simulink model "mrefrobotarm_modified_previous_y_error_previous_u"  (R2018b)
settings: Solver=FixedStepAuto  StartTime=0.0  StopTime=60  RelTol=1e-3  AbsTol=1e-6
undefined symbols (not defined in the file or in its folder): now, sfunxy2, simin
libraries: neural x368, simulink x1
(part 3 of 10)

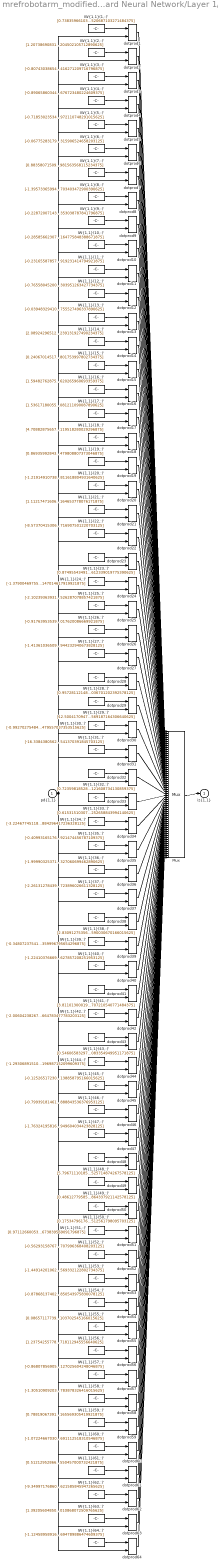
== system mrefrobotarm_modified_previous_y_error_previous_u/Feed-Forward Neural Network/Layer 1/IW{1,1} ==
  "pd{1,1}" : Inport  PortDimensions=7
      mask Display: e = 0.06;c1 = [120 230 180]/255;c2 = ([120 230 180]+0)/(256+128);c3 = ([120 230 180]+128)/(256+128);patch([0 1 1 0],[0 0 1 1],c1);patch([0 1 1 1-e 1-e 0+e],[0 0 1 1-e 0+e 0+e],c2);patch([0 0 1 1-e 0+e 0+e],[0 1 1 1-e 1-e 0+e],c3);plot([0 1 1 0 0],[0 0 1 1 0]);
  "IW{1,1}(1,:)'" : Constant  Value=[0.73835966103695149787000673313741572201251983642578125;-0.94961190463521660820589431750704534351825714111328125;1.6035911924959707075544201870798133313655853271484375;1.2440476828636082284873509706812910735607147216796875;-1.3632517507492050157225094153545796871185302734375;-0.5284581869871158854579107355675660073757171630859375;0.17161240081002249180386343141435645520687103271484375]
      mask Display: e = 0.06;c1 = [120 150 230]/255;c2 = ([120 150 230]+0)/383;c3 = ([120 150 230]+128)/383;patch([0 1 1 0],[0 0 1 1],c1);patch([0 1 1 1-e 1-e 0+e],[0 0 1 1-e 0+e 0+e],c2);patch([0 0 1 1-e 0+e 0+e],[0 1 1 1-e 1-e 0+e],c3);plot([0 1 1 0 0],[0 0 1 1 0]);disp('Weights');
  "IW{1,1}(10,:)'" : Constant  Value=[-0.285856623070984305901021116369520314037799835205078125;0.2344776406677883950901986054304870776832103729248046875;-1.315520776721690321409141688491217792034149169921875;1.074880530465292860498038862715475261211395263671875;-2.319666095832283669864182229503057897090911865234375;0.6986740963338966547979680399294011294841766357421875;-0.300490225799896648606335247677634470164775848388671875]
      mask Display: e = 0.06;c1 = [120 150 230]/255;c2 = ([120 150 230]+0)/383;c3 = ([120 150 230]+128)/383;patch([0 1 1 0],[0 0 1 1],c1);patch([0 1 1 1-e 1-e 0+e],[0 0 1 1-e 0+e 0+e],c2);patch([0 0 1 1-e 0+e 0+e],[0 1 1 1-e 1-e 0+e],c3);plot([0 1 1 0 0],[0 0 1 1 0]);disp('Weights');
  "IW{1,1}(11,:)'" : Constant  Value=[-0.2316558785704640743841054018048453144729137420654296875;0.69436199539330900609712671212037093937397003173828125;0.0092057493650668266449432763920412980951368808746337890625;1.1913003539647768480591594197903759777545928955078125;0.329665431400123776217725435344618745148181915283203125;-0.03705915414620364334297164532472379505634307861328125;-2.367396266890927858383975035394541919231414794921875]
      mask Display: e = 0.06;c1 = [120 150 230]/255;c2 = ([120 150 230]+0)/383;c3 = ([120 150 230]+128)/383;patch([0 1 1 0],[0 0 1 1],c1);patch([0 1 1 1-e 1-e 0+e],[0 0 1 1-e 0+e 0+e],c2);patch([0 0 1 1-e 0+e 0+e],[0 1 1 1-e 1-e 0+e],c3);plot([0 1 1 0 0],[0 0 1 1 0]);disp('Weights');
  "IW{1,1}(12,:)'" : Constant  Value=[-0.76558045200224367210495302060735411942005157470703125;-1.3880666042352911571100548826507292687892913818359375;1.240281466247820763015852207900024950504302978515625;-0.0943438152588715051027890012846910394728183746337890625;-1.1016339629113909293067763428553007543087005615234375;0.77645097802456730651243788088322617113590240478515625;1.0157545017459932434888969510211609303951263427734375]
      mask Display: e = 0.06;c1 = [120 150 230]/255;c2 = ([120 150 230]+0)/383;c3 = ([120 150 230]+128)/383;patch([0 1 1 0],[0 0 1 1],c1);patch([0 1 1 1-e 1-e 0+e],[0 0 1 1-e 0+e 0+e],c2);patch([0 0 1 1-e 0+e 0+e],[0 1 1 1-e 1-e 0+e],c3);plot([0 1 1 0 0],[0 0 1 1 0]);disp('Weights');
  "IW{1,1}(13,:)'" : Constant  Value=[-0.0394832941047644492282842065833392553031444549560546875;0.2683433283804415037110402408870868384838104248046875;-1.9772412570219646266167501380550675094127655029296875;-1.3369533766644858818750662976526655256748199462890625;0.383848968826891734362760644216905348002910614013671875;-0.82866232479277546207896421037730760872364044189453125;-0.71448374375757206511394770132028497755527496337890625]
      mask Display: e = 0.06;c1 = [120 150 230]/255;c2 = ([120 150 230]+0)/383;c3 = ([120 150 230]+128)/383;patch([0 1 1 0],[0 0 1 1],c1);patch([0 1 1 1-e 1-e 0+e],[0 0 1 1-e 0+e 0+e],c2);patch([0 0 1 1-e 0+e 0+e],[0 1 1 1-e 1-e 0+e],c3);plot([0 1 1 0 0],[0 0 1 1 0]);disp('Weights');
  "IW{1,1}(14,:)'" : Constant  Value=[2.089242965128133899810336515656672418117523193359375;1.0583956137306387290664133615791797637939453125;1.2221961841086137479095441449317149817943572998046875;-0.9640381765065815233839430220541544258594512939453125;2.007169466431919513382808872847817838191986083984375;-0.005116273422281165071667796695464858203195035457611083984375;0.5419457531010729578468954059644602239131927490234375]
      mask Display: e = 0.06;c1 = [120 150 230]/255;c2 = ([120 150 230]+0)/383;c3 = ([120 150 230]+128)/383;patch([0 1 1 0],[0 0 1 1],c1);patch([0 1 1 1-e 1-e 0+e],[0 0 1 1-e 0+e 0+e],c2);patch([0 0 1 1-e 0+e 0+e],[0 1 1 1-e 1-e 0+e],c3);plot([0 1 1 0 0],[0 0 1 1 0]);disp('Weights');
  "IW{1,1}(15,:)'" : Constant  Value=[0.240670145172809435418770362957729957997798919677734375;-0.37262437066721532108459769006003625690937042236328125;0.7519452971248181682994982111267745494842529296875;-0.43618047326959208387364697045995853841304779052734375;-2.164127657796442338877795918961055576801300048828125;-1.4690578945890966355847240265575237572193145751953125;1.03041595327624602163041345193050801753997802734375]
      mask Display: e = 0.06;c1 = [120 150 230]/255;c2 = ([120 150 230]+0)/383;c3 = ([120 150 230]+128)/383;patch([0 1 1 0],[0 0 1 1],c1);patch([0 1 1 1-e 1-e 0+e],[0 0 1 1-e 0+e 0+e],c2);patch([0 0 1 1-e 0+e 0+e],[0 1 1 1-e 1-e 0+e],c3);plot([0 1 1 0 0],[0 0 1 1 0]);disp('Weights');
  "IW{1,1}(16,:)'" : Constant  Value=[1.594827628756812831767319948994554579257965087890625;-0.409790418491936481171222794728237204253673553466796875;0.5354336553033169909809885211871005594730377197265625;0.293245297642927560399783715183730237185955047607421875;-1.1159358132358245807580487962695769965648651123046875;0.6919927373218188737524769749143160879611968994140625;-1.12512451883200181868005529395304620265960693359375]
      mask Display: e = 0.06;c1 = [120 150 230]/255;c2 = ([120 150 230]+0)/383;c3 = ([120 150 230]+128)/383;patch([0 1 1 0],[0 0 1 1],c1);patch([0 1 1 1-e 1-e 0+e],[0 0 1 1-e 0+e 0+e],c2);patch([0 0 1 1-e 0+e 0+e],[0 1 1 1-e 1-e 0+e],c3);plot([0 1 1 0 0],[0 0 1 1 0]);disp('Weights');
  "IW{1,1}(17,:)'" : Constant  Value=[1.536171800559593680901571133290417492389678955078125;0.044760026132134471399393049750869977287948131561279296875;0.6869129687880015655565557608497329056262969970703125;0.475311403464723836176375471040955744683742523193359375;0.429599864159958599874045148681034334003925323486328125;2.369256087953004907831200398504734039306640625;0.80062373149870647015546865077340044081211090087890625]
      mask Display: e = 0.06;c1 = [120 150 230]/255;c2 = ([120 150 230]+0)/383;c3 = ([120 150 230]+128)/383;patch([0 1 1 0],[0 0 1 1],c1);patch([0 1 1 1-e 1-e 0+e],[0 0 1 1-e 0+e 0+e],c2);patch([0 0 1 1-e 0+e 0+e],[0 1 1 1-e 1-e 0+e],c3);plot([0 1 1 0 0],[0 0 1 1 0]);disp('Weights');
  "IW{1,1}(18,:)'" : Constant  Value=[4.70882875657937471913783156196586787700653076171875;1.0182941971839178929570834952755831182003021240234375;-0.29646960125124144358466082849190570414066314697265625;-2.63562093522858020833155023865401744842529296875;1.25983914696097176744160606176592409610748291015625;0.8392764608202714082807460727053694427013397216796875;0.38937859950317121882079618444549851119518280029296875]
      mask Display: e = 0.06;c1 = [120 150 230]/255;c2 = ([120 150 230]+0)/383;c3 = ([120 150 230]+128)/383;patch([0 1 1 0],[0 0 1 1],c1);patch([0 1 1 1-e 1-e 0+e],[0 0 1 1-e 0+e 0+e],c2);patch([0 0 1 1-e 0+e 0+e],[0 1 1 1-e 1-e 0+e],c3);plot([0 1 1 0 0],[0 0 1 1 0]);disp('Weights');
  "IW{1,1}(19,:)'" : Constant  Value=[0.86935992843650655714782260474748909473419189453125;1.2256376561587603024605641621747054159641265869140625;-0.74215457486800462394427313483902253210544586181640625;-0.749309744190128856899946185876615345478057861328125;-1.0295529762959614306083722112816758453845977783203125;-1.6497508162831613365284511019126512110233306884765625;0.21325656607528908903503861438366584479808807373046875]
      mask Display: e = 0.06;c1 = [120 150 230]/255;c2 = ([120 150 230]+0)/383;c3 = ([120 150 230]+128)/383;patch([0 1 1 0],[0 0 1 1],c1);patch([0 1 1 1-e 1-e 0+e],[0 0 1 1-e 0+e 0+e],c2);patch([0 0 1 1-e 0+e 0+e],[0 1 1 1-e 1-e 0+e],c3);plot([0 1 1 0 0],[0 0 1 1 0]);disp('Weights');
  "IW{1,1}(2,:)'" : Constant  Value=[1.207386908319982854465024502133019268512725830078125;0.60142973756388518058457748338696546852588653564453125;1.4282422078554113387127699752454645931720733642578125;1.129810122922250581467551455716602504253387451171875;0.52929546216326650576178280971362255513668060302734375;-0.521340349014109083469747929484583437442779541015625;-0.57746032918438638947833396741771139204502105712890625]
      mask Display: e = 0.06;c1 = [120 150 230]/255;c2 = ([120 150 230]+0)/383;c3 = ([120 150 230]+128)/383;patch([0 1 1 0],[0 0 1 1],c1);patch([0 1 1 1-e 1-e 0+e],[0 0 1 1-e 0+e 0+e],c2);patch([0 0 1 1-e 0+e 0+e],[0 1 1 1-e 1-e 0+e],c3);plot([0 1 1 0 0],[0 0 1 1 0]);disp('Weights');
  "IW{1,1}(20,:)'" : Constant  Value=[-1.2191491073873752526424141251482069492340087890625;0.292212917054135157268746070258202962577342987060546875;-0.62705777055215461412984723210684023797512054443359375;1.34344981494831916535304117132909595966339111328125;-0.466225081988995981863155293467571027576923370361328125;1.16396408978602483585973459412343800067901611328125;1.0600774509352677288376298747607506811618804931640625]
      mask Display: e = 0.06;c1 = [120 150 230]/255;c2 = ([120 150 230]+0)/383;c3 = ([120 150 230]+128)/383;patch([0 1 1 0],[0 0 1 1],c1);patch([0 1 1 1-e 1-e 0+e],[0 0 1 1-e 0+e 0+e],c2);patch([0 0 1 1-e 0+e 0+e],[0 1 1 1-e 1-e 0+e],c3);plot([0 1 1 0 0],[0 0 1 1 0]);disp('Weights');
  "IW{1,1}(21,:)'" : Constant  Value=[1.1121747160646184848786788279539905488491058349609375;-0.60810994087790193329823296153335832059383392333984375;0.90343241269697427409113288376829586923122406005859375;0.340373330006717267348648192637483589351177215576171875;-1.1890993364047857117071771426708437502384185791015625;1.9229246604893981409389880354865454137325286865234375;-0.5950707485470914104297435187618248164653778076171875]
      mask Display: e = 0.06;c1 = [120 150 230]/255;c2 = ([120 150 230]+0)/383;c3 = ([120 150 230]+128)/383;patch([0 1 1 0],[0 0 1 1],c1);patch([0 1 1 1-e 1-e 0+e],[0 0 1 1-e 0+e 0+e],c2);patch([0 0 1 1-e 0+e 0+e],[0 1 1 1-e 1-e 0+e],c3);plot([0 1 1 0 0],[0 0 1 1 0]);disp('Weights');
  "IW{1,1}(22,:)'" : Constant  Value=[-8.57370415306336752792049082927405834197998046875;4.0171564439012374947424177662469446659088134765625;2.0196425514487454933032495318911969661712646484375;-0.0038727846207056125515943989512379630468785762786865234375;0.17380867661798760082092485390603542327880859375;-0.895012208914945706084154153359122574329376220703125;-1.240911378886007998545437658322043716907501220703125]
      mask Display: e = 0.06;c1 = [120 150 230]/255;c2 = ([120 150 230]+0)/383;c3 = ([120 150 230]+128)/383;patch([0 1 1 0],[0 0 1 1],c1);patch([0 1 1 1-e 1-e 0+e],[0 0 1 1-e 0+e 0+e],c2);patch([0 0 1 1-e 0+e 0+e],[0 1 1 1-e 1-e 0+e],c3);plot([0 1 1 0 0],[0 0 1 1 0]);disp('Weights');
  "IW{1,1}(23,:)'" : Constant  Value=[0.87495543491740790376098857450415380299091339111328125;-1.548464555412043086590756502118892967700958251953125;1.159091997448419508742745165363885462284088134765625;0.69503432512084539762753365721437148749828338623046875;0.359854826398857741143189059584983624517917633056640625;-0.626666123302821898022330060484819114208221435546875;-0.419306439460687130349469953216612339019775390625]
      mask Display: e = 0.06;c1 = [120 150 230]/255;c2 = ([120 150 230]+0)/383;c3 = ([120 150 230]+128)/383;patch([0 1 1 0],[0 0 1 1],c1);patch([0 1 1 1-e 1-e 0+e],[0 0 1 1-e 0+e 0+e],c2);patch([0 0 1 1-e 0+e 0+e],[0 1 1 1-e 1-e 0+e],c3);plot([0 1 1 0 0],[0 0 1 1 0]);disp('Weights');
  "IW{1,1}(24,:)'" : Constant  Value=[-1.3790046975524656858169691986404359340667724609375;1.1977931691528158619775012994068674743175506591796875;0.8600690763459706289495443343184888362884521484375;-1.33526003303544538169944644323550164699554443359375;1.2562328890788150292934233220876194536685943603515625;-0.5055283895922257908495112133095972239971160888671875;-0.2278459789949866809433132175399805419147014617919921875]
      mask Display: e = 0.06;c1 = [120 150 230]/255;c2 = ([120 150 230]+0)/383;c3 = ([120 150 230]+128)/383;patch([0 1 1 0],[0 0 1 1],c1);patch([0 1 1 1-e 1-e 0+e],[0 0 1 1-e 0+e 0+e],c2);patch([0 0 1 1-e 0+e 0+e],[0 1 1 1-e 1-e 0+e],c3);plot([0 1 1 0 0],[0 0 1 1 0]);disp('Weights');
  "IW{1,1}(25,:)'" : Constant  Value=[-2.102393639314213746871473631472326815128326416015625;-3.76389751408084283212929221917875111103057861328125;2.078769576669774910016030844417400658130645751953125;0.38950132659974967541671730941743589937686920166015625;-4.26745758288289689375005764304660260677337646484375;0.5340540555107826659053671392030082643032073974609375;1.8287537538784099933053539643879048526287078857421875]
      mask Display: e = 0.06;c1 = [120 150 230]/255;c2 = ([120 150 230]+0)/383;c3 = ([120 150 230]+128)/383;patch([0 1 1 0],[0 0 1 1],c1);patch([0 1 1 1-e 1-e 0+e],[0 0 1 1-e 0+e 0+e],c2);patch([0 0 1 1-e 0+e 0+e],[0 1 1 1-e 1-e 0+e],c3);plot([0 1 1 0 0],[0 0 1 1 0]);disp('Weights');
  "IW{1,1}(26,:)'" : Constant  Value=[-0.9176395353965032253285016849986277520656585693359375;-0.04458878245606212598062256802222691476345062255859375;1.3530432976563921965151848780806176364421844482421875;0.02686983344273292939607955531755578704178333282470703125;-2.705305218699319613762099834275431931018829345703125;0.73214756050264251374670720906578935682773590087890625;0.62440621397350504206968935250188224017620086669921875]
      mask Display: e = 0.06;c1 = [120 150 230]/255;c2 = ([120 150 230]+0)/383;c3 = ([120 150 230]+128)/383;patch([0 1 1 0],[0 0 1 1],c1);patch([0 1 1 1-e 1-e 0+e],[0 0 1 1-e 0+e 0+e],c2);patch([0 0 1 1-e 0+e 0+e],[0 1 1 1-e 1-e 0+e],c3);plot([0 1 1 0 0],[0 0 1 1 0]);disp('Weights');
  "IW{1,1}(27,:)'" : Constant  Value=[-1.41361036509884119283242398523725569248199462890625;-0.2148998090111946812630350223116693086922168731689453125;-0.88851175150081640463639587323996238410472869873046875;0.445203605566461158016267063430859707295894622802734375;0.356930601207742059788330379888066090643405914306640625;2.115478385494487412188391317613422870635986328125;1.68742965335181782648987791617400944232940673828125]
      mask Display: e = 0.06;c1 = [120 150 230]/255;c2 = ([120 150 230]+0)/383;c3 = ([120 150 230]+128)/383;patch([0 1 1 0],[0 0 1 1],c1);patch([0 1 1 1-e 1-e 0+e],[0 0 1 1-e 0+e 0+e],c2);patch([0 0 1 1-e 0+e 0+e],[0 1 1 1-e 1-e 0+e],c3);plot([0 1 1 0 0],[0 0 1 1 0]);disp('Weights');
  "IW{1,1}(28,:)'" : Constant  Value=[0.9572811214803549351159972502500750124454498291015625;-0.9448130506895486835361452904180623590946197509765625;-1.843363693261503843956461423658765852451324462890625;-0.09870357560995070278497820481788949109613895416259765625;-0.432231125687960238135332247111364267766475677490234375;1.5519178923840619699348053472931496798992156982421875;1.362051502548276449289232914452441036701202392578125]
      mask Display: e = 0.06;c1 = [120 150 230]/255;c2 = ([120 150 230]+0)/383;c3 = ([120 150 230]+128)/383;patch([0 1 1 0],[0 0 1 1],c1);patch([0 1 1 1-e 1-e 0+e],[0 0 1 1-e 0+e 0+e],c2);patch([0 0 1 1-e 0+e 0+e],[0 1 1 1-e 1-e 0+e],c3);plot([0 1 1 0 0],[0 0 1 1 0]);disp('Weights');
  "IW{1,1}(29,:)'" : Constant  Value=[12.5004170947519224199595555546693503856658935546875;1.7035842613993403826810890677734278142452239990234375;-4.5262638802356196521259334986098110675811767578125;-3.2918155677113301038616555160842835903167724609375;0.0989294068375679014337720218463800847530364990234375;1.7539877591714070348416498745791614055633544921875;-0.53021136566533899614483971163281239569187164306640625]
      mask Display: e = 0.06;c1 = [120 150 230]/255;c2 = ([120 150 230]+0)/383;c3 = ([120 150 230]+128)/383;patch([0 1 1 0],[0 0 1 1],c1);patch([0 1 1 1-e 1-e 0+e],[0 0 1 1-e 0+e 0+e],c2);patch([0 0 1 1-e 0+e 0+e],[0 1 1 1-e 1-e 0+e],c3);plot([0 1 1 0 0],[0 0 1 1 0]);disp('Weights');
  "IW{1,1}(3,:)'" : Constant  Value=[-0.80743038654165977252574748490587808191776275634765625;1.48604428772479391085425959317944943904876708984375;1.514383091511012136010094764060340821743011474609375;0.93867883654444217444989817522582598030567169189453125;-0.043116312200369509566311165826846263371407985687255859375;1.16577600469918873926644664607010781764984130859375;-0.06996023283199341580296248821468907408416271209716796875]
      mask Display: e = 0.06;c1 = [120 150 230]/255;c2 = ([120 150 230]+0)/383;c3 = ([120 150 230]+128)/383;patch([0 1 1 0],[0 0 1 1],c1);patch([0 1 1 1-e 1-e 0+e],[0 0 1 1-e 0+e 0+e],c2);patch([0 0 1 1-e 0+e 0+e],[0 1 1 1-e 1-e 0+e],c3);plot([0 1 1 0 0],[0 0 1 1 0]);disp('Weights');
  "IW{1,1}(30,:)'" : Constant  Value=[-0.992702754844593027172550137038342654705047607421875;0.477233746452680296368242807147908024489879608154296875;-1.0764384567135694137363088884740136563777923583984375;-1.2150756811348990549248583192820660769939422607421875;0.7911923672672009910655788189615122973918914794921875;-1.1658964213197278159128700281144119799137115478515625;0.2432016545416344488472759621799923479557037353515625]
      mask Display: e = 0.06;c1 = [120 150 230]/255;c2 = ([120 150 230]+0)/383;c3 = ([120 150 230]+128)/383;patch([0 1 1 0],[0 0 1 1],c1);patch([0 1 1 1-e 1-e 0+e],[0 0 1 1-e 0+e 0+e],c2);patch([0 0 1 1-e 0+e 0+e],[0 1 1 1-e 1-e 0+e],c3);plot([0 1 1 0 0],[0 0 1 1 0]);disp('Weights');
  "IW{1,1}(31,:)'" : Constant  Value=[-16.338438056299370515489499666728079319000244140625;5.677906950832653620864221011288464069366455078125;1.257177629119180295447222306393086910247802734375;3.084543449354010480334409294300712645053863525390625;1.93049991449494573458878221572376787662506103515625;-2.08848821422302943773274819250218570232391357421875;-0.96472404387054322416616969348979182541370391845703125]
      mask Display: e = 0.06;c1 = [120 150 230]/255;c2 = ([120 150 230]+0)/383;c3 = ([120 150 230]+128)/383;patch([0 1 1 0],[0 0 1 1],c1);patch([0 1 1 1-e 1-e 0+e],[0 0 1 1-e 0+e 0+e],c2);patch([0 0 1 1-e 0+e 0+e],[0 1 1 1-e 1-e 0+e],c3);plot([0 1 1 0 0],[0 0 1 1 0]);disp('Weights');
  "IW{1,1}(32,:)'" : Constant  Value=[0.72359818528620045707810959356720559298992156982421875;-1.6440003314616358220945357970776967704296112060546875;-0.83050079319534830801785574294626712799072265625;0.27573713468012128746664757272810675203800201416015625;0.223506350461608604973662295378744602203369140625;-1.95819542324606121752594845020212233066558837890625;-2.0879808382233644437064867815934121608734130859375]
      mask Display: e = 0.06;c1 = [120 150 230]/255;c2 = ([120 150 230]+0)/383;c3 = ([120 150 230]+128)/383;patch([0 1 1 0],[0 0 1 1],c1);patch([0 1 1 1-e 1-e 0+e],[0 0 1 1-e 0+e 0+e],c2);patch([0 0 1 1-e 0+e 0+e],[0 1 1 1-e 1-e 0+e],c3);plot([0 1 1 0 0],[0 0 1 1 0]);disp('Weights');
  "IW{1,1}(33,:)'" : Constant  Value=[0.6153151030709864688361676599015481770038604736328125;0.6691272401310477402347487441147677600383758544921875;-0.72784086034873485271390336492913775146007537841796875;-1.120378191299657988366789140854962170124053955078125;-0.51930559479426141589186727287597022950649261474609375;0.56780815440402976346234709126292727887630462646484375;-1.6152046873764975831733181621530093252658843994140625]
      mask Display: e = 0.06;c1 = [120 150 230]/255;c2 = ([120 150 230]+0)/383;c3 = ([120 150 230]+128)/383;patch([0 1 1 0],[0 0 1 1],c1);patch([0 1 1 1-e 1-e 0+e],[0 0 1 1-e 0+e 0+e],c2);patch([0 0 1 1-e 0+e 0+e],[0 1 1 1-e 1-e 0+e],c3);plot([0 1 1 0 0],[0 0 1 1 0]);disp('Weights');
  "IW{1,1}(34,:)'" : Constant  Value=[-3.22467745118568505091616316349245607852935791015625;2.8959677209624832272538696997798979282379150390625;0.77094836502237018560634851382928900420665740966796875;-2.821540095988474217136854349519126117229461669921875;-1.5536333997586166955073849749169312417507171630859375;1.0360973498748424770354858992504887282848358154296875;0.97325103763728748607064744646777398884296417236328125]
      mask Display: e = 0.06;c1 = [120 150 230]/255;c2 = ([120 150 230]+0)/383;c3 = ([120 150 230]+128)/383;patch([0 1 1 0],[0 0 1 1],c1);patch([0 1 1 1-e 1-e 0+e],[0 0 1 1-e 0+e 0+e],c2);patch([0 0 1 1-e 0+e 0+e],[0 1 1 1-e 1-e 0+e],c3);plot([0 1 1 0 0],[0 0 1 1 0]);disp('Weights');
  "IW{1,1}(35,:)'" : Constant  Value=[-0.40993165176265533578003896764130331575870513916015625;-2.33898377229580223257698889938183128833770751953125;0.32897348394588943332195185575983487069606781005859375;-0.56615619560323582337701964206644333899021148681640625;-0.41003241083886809992264943502959795296192169189453125;1.2140401389446784374825938357389532029628753662109375;-0.85422786927035010418052252134657464921474456787109375]
      mask Display: e = 0.06;c1 = [120 150 230]/255;c2 = ([120 150 230]+0)/383;c3 = ([120 150 230]+128)/383;patch([0 1 1 0],[0 0 1 1],c1);patch([0 1 1 1-e 1-e 0+e],[0 0 1 1-e 0+e 0+e],c2);patch([0 0 1 1-e 0+e 0+e],[0 1 1 1-e 1-e 0+e],c3);plot([0 1 1 0 0],[0 0 1 1 0]);disp('Weights');
  "IW{1,1}(36,:)'" : Constant  Value=[-1.9999032537141001597547074197791516780853271484375;-2.974276201114873341424527097842656075954437255859375;-1.7007569264815598497619930640212260186672210693359375;2.149370754668828542577330154017545282840728759765625;-0.09993625247978608905352615465744747780263423919677734375;-0.53677678761069558266427748094429261982440948486328125;-0.22378503182603604049205614501261152327060699462890625]
      mask Display: e = 0.06;c1 = [120 150 230]/255;c2 = ([120 150 230]+0)/383;c3 = ([120 150 230]+128)/383;patch([0 1 1 0],[0 0 1 1],c1);patch([0 1 1 1-e 1-e 0+e],[0 0 1 1-e 0+e 0+e],c2);patch([0 0 1 1-e 0+e 0+e],[0 1 1 1-e 1-e 0+e],c3);plot([0 1 1 0 0],[0 0 1 1 0]);disp('Weights');
  "IW{1,1}(37,:)'" : Constant  Value=[-2.261312784396285024968165089376270771026611328125;-1.68433878042118667650584029615856707096099853515625;0.92988448033931081493363990375655703246593475341796875;-0.08506420369932309044624929583733319304883480072021484375;2.1538362566721378499323691357858479022979736328125;-1.9027585984741450797486095325439237058162689208984375;-1.091765486344769886528638380696065723896026611328125]
      mask Display: e = 0.06;c1 = [120 150 230]/255;c2 = ([120 150 230]+0)/383;c3 = ([120 150 230]+128)/383;patch([0 1 1 0],[0 0 1 1],c1);patch([0 1 1 1-e 1-e 0+e],[0 0 1 1-e 0+e 0+e],c2);patch([0 0 1 1-e 0+e 0+e],[0 1 1 1-e 1-e 0+e],c3);plot([0 1 1 0 0],[0 0 1 1 0]);disp('Weights');
  "IW{1,1}(38,:)'" : Constant  Value=[2.830912753563269657064438433735631406307220458984375;-0.10314084738627983528491682818639674223959445953369140625;-1.0692129299568013944821132099605165421962738037109375;-1.98670442322062523743397832731716334819793701171875;-0.94562071413735726554961047440883703529834747314453125;-0.78961674023875005890005240871687419712543487548828125;0.70458382474041825194177590674371458590030670166015625]
      mask Display: e = 0.06;c1 = [120 150 230]/255;c2 = ([120 150 230]+0)/383;c3 = ([120 150 230]+128)/383;patch([0 1 1 0],[0 0 1 1],c1);patch([0 1 1 1-e 1-e 0+e],[0 0 1 1-e 0+e 0+e],c2);patch([0 0 1 1-e 0+e 0+e],[0 1 1 1-e 1-e 0+e],c3);plot([0 1 1 0 0],[0 0 1 1 0]);disp('Weights');
  "IW{1,1}(39,:)'" : Constant  Value=[-0.348072375411236978326456892318674363195896148681640625;-1.6510457560732707538164731886354275047779083251953125;-1.2916493330084086732512105299974791705608367919921875;1.042360874067343790017048377194441854953765869140625;0.1427982759597591078115641494150622747838497161865234375;-1.2845046490448479570289919138303957879543304443359375;1.5124340845957024992429751364397816359996795654296875]
      mask Display: e = 0.06;c1 = [120 150 230]/255;c2 = ([120 150 230]+0)/383;c3 = ([120 150 230]+128)/383;patch([0 1 1 0],[0 0 1 1],c1);patch([0 1 1 1-e 1-e 0+e],[0 0 1 1-e 0+e 0+e],c2);patch([0 0 1 1-e 0+e 0+e],[0 1 1 1-e 1-e 0+e],c3);plot([0 1 1 0 0],[0 0 1 1 0]);disp('Weights');
  "IW{1,1}(4,:)'" : Constant  Value=[-0.89065860344844749452164478498161770403385162353515625;-1.2324761697914368152595443461905233561992645263671875;-0.96599148156176972701558725020731799304485321044921875;0.2017190712792409357234646449796855449676513671875;0.69131736008931865544724360006512142717838287353515625;-1.715661921858600447166054436820559203624725341796875;0.7329642167055145929310810970491729676723480224609375]
      mask Display: e = 0.06;c1 = [120 150 230]/255;c2 = ([120 150 230]+0)/383;c3 = ([120 150 230]+128)/383;patch([0 1 1 0],[0 0 1 1],c1);patch([0 1 1 1-e 1-e 0+e],[0 0 1 1-e 0+e 0+e],c2);patch([0 0 1 1-e 0+e 0+e],[0 1 1 1-e 1-e 0+e],c3);plot([0 1 1 0 0],[0 0 1 1 0]);disp('Weights');
  "IW{1,1}(40,:)'" : Constant  Value=[-1.224103766692140826677359655150212347507476806640625;-1.0366503183705189083951836437336169183254241943359375;-0.5230620278335227357757730715093202888965606689453125;0.469679422742529439904757282420177944004535675048828125;-1.7855954655395096519754360997467301785945892333984375;-1.733929619164484403626147468457929790019989013671875;0.8116215075814612323057417597738094627857208251953125]
      mask Display: e = 0.06;c1 = [120 150 230]/255;c2 = ([120 150 230]+0)/383;c3 = ([120 150 230]+128)/383;patch([0 1 1 0],[0 0 1 1],c1);patch([0 1 1 1-e 1-e 0+e],[0 0 1 1-e 0+e 0+e],c2);patch([0 0 1 1-e 0+e 0+e],[0 1 1 1-e 1-e 0+e],c3);plot([0 1 1 0 0],[0 0 1 1 0]);disp('Weights');
  "IW{1,1}(41,:)'" : Constant  Value=[3.811013000198275602059538869070820510387420654296875;0.5832783973862503135165979983867146074771881103515625;0.255772029265343869841586865732097066938877105712890625;-1.5158757185097153641351042097085155546665191650390625;-1.7725277268672356978385096226702444255352020263671875;1.5701810780917870857820162200368940830230712890625;0.81793887234063633595582132329582236707210540771484375]
      mask Display: e = 0.06;c1 = [120 150 230]/255;c2 = ([120 150 230]+0)/383;c3 = ([120 150 230]+128)/383;patch([0 1 1 0],[0 0 1 1],c1);patch([0 1 1 1-e 1-e 0+e],[0 0 1 1-e 0+e 0+e],c2);patch([0 0 1 1-e 0+e 0+e],[0 1 1 1-e 1-e 0+e],c3);plot([0 1 1 0 0],[0 0 1 1 0]);disp('Weights');
  "IW{1,1}(42,:)'" : Constant  Value=[-2.006042382672766688500587406451813876628875732421875;1.0413470547606602512047402342432178556919097900390625;-1.6362398327674068099213400273583829402923583984375;0.62619619818024074842099935267469845712184906005859375;-1.4551768832123423980107190800481475889682769775390625;-0.1490826525180633244094252631839481182396411895751953125;-0.38461134741321967300820006130379624664783477783203125]
      mask Display: e = 0.06;c1 = [120 150 230]/255;c2 = ([120 150 230]+0)/383;c3 = ([120 150 230]+128)/383;patch([0 1 1 0],[0 0 1 1],c1);patch([0 1 1 1-e 1-e 0+e],[0 0 1 1-e 0+e 0+e],c2);patch([0 0 1 1-e 0+e 0+e],[0 1 1 1-e 1-e 0+e],c3);plot([0 1 1 0 0],[0 0 1 1 0]);disp('Weights');
  "IW{1,1}(43,:)'" : Constant  Value=[0.5460658329776328923088613009895198047161102294921875;-0.94530550980993510723493500336189754307270050048828125;1.70665652034300752148965329979546368122100830078125;0.96956623158008647944683389141573570668697357177734375;0.3589279855235745220198850802262313663959503173828125;-1.1420047056002007312969226404675282537937164306640625;1.132817899182256393686429873923771083354949951171875]
      mask Display: e = 0.06;c1 = [120 150 230]/255;c2 = ([120 150 230]+0)/383;c3 = ([120 150 230]+128)/383;patch([0 1 1 0],[0 0 1 1],c1);patch([0 1 1 1-e 1-e 0+e],[0 0 1 1-e 0+e 0+e],c2);patch([0 0 1 1-e 0+e 0+e],[0 1 1 1-e 1-e 0+e],c3);plot([0 1 1 0 0],[0 0 1 1 0]);disp('Weights');
  "IW{1,1}(44,:)'" : Constant  Value=[-1.2930689151046041995840596428024582564830780029296875;-0.56249698171321116380028115599998272955417633056640625;1.32754142274804731727044782019220292568206787109375;0.74378133140686986113365719575085677206516265869140625;-1.23374094380344079269207213656045496463775634765625;-1.0689189038876143467149404386873356997966766357421875;0.374826487480591941103824638048536144196987152099609375]
      mask Display: e = 0.06;c1 = [120 150 230]/255;c2 = ([120 150 230]+0)/383;c3 = ([120 150 230]+128)/383;patch([0 1 1 0],[0 0 1 1],c1);patch([0 1 1 1-e 1-e 0+e],[0 0 1 1-e 0+e 0+e],c2);patch([0 0 1 1-e 0+e 0+e],[0 1 1 1-e 1-e 0+e],c3);plot([0 1 1 0 0],[0 0 1 1 0]);disp('Weights');
  "IW{1,1}(45,:)'" : Constant  Value=[-0.125265172307327643519414550610235892236232757568359375;-1.2979706658467675683965580901713110506534576416015625;-1.2591143708802052803008564296760596334934234619140625;-1.1810024297842882656794927243026904761791229248046875;0.9690025756252274025115411859587766230106353759765625;0.775011346863422989628134018857963383197784423828125;0.342495238331483931037979573375196196138858795166015625]
      mask Display: e = 0.06;c1 = [120 150 230]/255;c2 = ([120 150 230]+0)/383;c3 = ([120 150 230]+128)/383;patch([0 1 1 0],[0 0 1 1],c1);patch([0 1 1 1-e 1-e 0+e],[0 0 1 1-e 0+e 0+e],c2);patch([0 0 1 1-e 0+e 0+e],[0 1 1 1-e 1-e 0+e],c3);plot([0 1 1 0 0],[0 0 1 1 0]);disp('Weights');
  "IW{1,1}(46,:)'" : Constant  Value=[-0.79939181461898367597740389101090840995311737060546875;-1.7847629951989552044011588805005885660648345947265625;-1.6422494523457071835537135484628379344940185546875;0.9750905072276481178050744347274303436279296875;-1.152209715275577917026339491712860763072967529296875;0.57577749736601047114703533225110732018947601318359375;-0.349444239740421214168719643566873855888843536376953125]
      mask Display: e = 0.06;c1 = [120 150 230]/255;c2 = ([120 150 230]+0)/383;c3 = ([120 150 230]+128)/383;patch([0 1 1 0],[0 0 1 1],c1);patch([0 1 1 1-e 1-e 0+e],[0 0 1 1-e 0+e 0+e],c2);patch([0 0 1 1-e 0+e 0+e],[0 1 1 1-e 1-e 0+e],c3);plot([0 1 1 0 0],[0 0 1 1 0]);disp('Weights');
  "IW{1,1}(47,:)'" : Constant  Value=[-1.7632419581677851727619099619914777576923370361328125;-2.088742863304435815052784164436161518096923828125;-0.314819559914206126283175990465679205954074859619140625;0.82991928825946670311708430745056830346584320068359375;-1.5806265425320786821572482949704863131046295166015625;1.0266114183991661423789309992571361362934112548828125;-0.0973938829209682055410013390428503043949604034423828125]
      mask Display: e = 0.06;c1 = [120 150 230]/255;c2 = ([120 150 230]+0)/383;c3 = ([120 150 230]+128)/383;patch([0 1 1 0],[0 0 1 1],c1);patch([0 1 1 1-e 1-e 0+e],[0 0 1 1-e 0+e 0+e],c2);patch([0 0 1 1-e 0+e 0+e],[0 1 1 1-e 1-e 0+e],c3);plot([0 1 1 0 0],[0 0 1 1 0]);disp('Weights');
  "IW{1,1}(48,:)'" : Constant  Value=[5.7967111018597705651700380258262157440185546875;-0.353441353033542460249094574464834295213222503662109375;-1.087621083945466526898826487013138830661773681640625;0.01317302208333899667114241793797191348858177661895751953125;-2.46855191535412021863749032490886747837066650390625;-0.01189689818004919900917837338738536345772445201873779296875;1.4291611738391403196857254442875273525714874267578125]
      mask Display: e = 0.06;c1 = [120 150 230]/255;c2 = ([120 150 230]+0)/383;c3 = ([120 150 230]+128)/383;patch([0 1 1 0],[0 0 1 1],c1);patch([0 1 1 1-e 1-e 0+e],[0 0 1 1-e 0+e 0+e],c2);patch([0 0 1 1-e 0+e 0+e],[0 1 1 1-e 1-e 0+e],c3);plot([0 1 1 0 0],[0 0 1 1 0]);disp('Weights');
  "IW{1,1}(49,:)'" : Constant  Value=[0.486127795858225242309202940305112861096858978271484375;0.746935613742211845789142898865975439548492431640625;1.577270606275454678524283735896460711956024169921875;1.4551426634219193356756250068428926169872283935546875;1.0852780717655947650968073503463529050350189208984375;0.29915236483236828934906270660576410591602325439453125;-0.40249497942065126654398454775218851864337921142578125]
      mask Display: e = 0.06;c1 = [120 150 230]/255;c2 = ([120 150 230]+0)/383;c3 = ([120 150 230]+128)/383;patch([0 1 1 0],[0 0 1 1],c1);patch([0 1 1 1-e 1-e 0+e],[0 0 1 1-e 0+e 0+e],c2);patch([0 0 1 1-e 0+e 0+e],[0 1 1 1-e 1-e 0+e],c3);plot([0 1 1 0 0],[0 0 1 1 0]);disp('Weights');
  "IW{1,1}(5,:)'" : Constant  Value=[-0.718530235345395507096100118360482156276702880859375;1.0522938916772464068571935058571398258209228515625;0.012909872082843769358628804866384598426520824432373046875;-1.75935310381194565110263283713720738887786865234375;0.62020539881142522364854130501043982803821563720703125;0.2252623906161243805268412643272313289344310760498046875;-1.132512354873596027715620948583818972110748291015625]
      mask Display: e = 0.06;c1 = [120 150 230]/255;c2 = ([120 150 230]+0)/383;c3 = ([120 150 230]+128)/383;patch([0 1 1 0],[0 0 1 1],c1);patch([0 1 1 1-e 1-e 0+e],[0 0 1 1-e 0+e 0+e],c2);patch([0 0 1 1-e 0+e 0+e],[0 1 1 1-e 1-e 0+e],c3);plot([0 1 1 0 0],[0 0 1 1 0]);disp('Weights');
  "IW{1,1}(50,:)'" : Constant  Value=[0.1753479617690769654103633001795969903469085693359375;1.8630588375631795816644853402976877987384796142578125;-2.24930435978582909939404999022372066974639892578125;-1.022563912494447446732692696969024837017059326171875;0.7920084208289974725403226329945027828216552734375;-1.634487470492640426300567924045026302337646484375;-0.533929514864834420251327173900790512561798095703125]
      mask Display: e = 0.06;c1 = [120 150 230]/255;c2 = ([120 150 230]+0)/383;c3 = ([120 150 230]+128)/383;patch([0 1 1 0],[0 0 1 1],c1);patch([0 1 1 1-e 1-e 0+e],[0 0 1 1-e 0+e 0+e],c2);patch([0 0 1 1-e 0+e 0+e],[0 1 1 1-e 1-e 0+e],c3);plot([0 1 1 0 0],[0 0 1 1 0]);disp('Weights');
  "IW{1,1}(51,:)'" : Constant  Value=[0.97112660053720756270223546380293555557727813720703125;-1.2031642341239867644020478110178373754024505615234375;-1.0209123550452974260593919098027981817722320556640625;1.190529033280860016219548924709670245647430419921875;0.06479861113599984234756590240067453123629093170166015625;0.252740880441116033683357500194688327610492706298828125;0.98618932561259942115583498889463953673839569091796875]
      mask Display: e = 0.06;c1 = [120 150 230]/255;c2 = ([120 150 230]+0)/383;c3 = ([120 150 230]+128)/383;patch([0 1 1 0],[0 0 1 1],c1);patch([0 1 1 1-e 1-e 0+e],[0 0 1 1-e 0+e 0+e],c2);patch([0 0 1 1-e 0+e 0+e],[0 1 1 1-e 1-e 0+e],c3);plot([0 1 1 0 0],[0 0 1 1 0]);disp('Weights');
  "IW{1,1}(52,:)'" : Constant  Value=[-0.56293158767136375342232668117503635585308074951171875;-0.98364077995051968361650551742059178650379180908203125;0.77290720047679040138888240107917226850986480712890625;0.71714923345493952755447253366583026945590972900390625;-1.9774234096473577437791391275823116302490234375;-1.3670014258104592475007166285649873316287994384765625;-1.2403558286757316864168387837707996368408203125]
      mask Display: e = 0.06;c1 = [120 150 230]/255;c2 = ([120 150 230]+0)/383;c3 = ([120 150 230]+128)/383;patch([0 1 1 0],[0 0 1 1],c1);patch([0 1 1 1-e 1-e 0+e],[0 0 1 1-e 0+e 0+e],c2);patch([0 0 1 1-e 0+e 0+e],[0 1 1 1-e 1-e 0+e],c3);plot([0 1 1 0 0],[0 0 1 1 0]);disp('Weights');
  "IW{1,1}(53,:)'" : Constant  Value=[-1.4491420106285197721973645457183010876178741455078125;1.3094456814424848545286295120604336261749267578125;-1.386646167148400277113751144497655332088470458984375;0.298468868056892155937731558879022486507892608642578125;-0.90017664137490827069854049113928340375423431396484375;-0.72217348977064410586734766184235922992229461669921875;0.1917842641023979888270645233205868862569332122802734375]
      mask Display: e = 0.06;c1 = [120 150 230]/255;c2 = ([120 150 230]+0)/383;c3 = ([120 150 230]+128)/383;patch([0 1 1 0],[0 0 1 1],c1);patch([0 1 1 1-e 1-e 0+e],[0 0 1 1-e 0+e 0+e],c2);patch([0 0 1 1-e 0+e 0+e],[0 1 1 1-e 1-e 0+e],c3);plot([0 1 1 0 0],[0 0 1 1 0]);disp('Weights');
  "IW{1,1}(54,:)'" : Constant  Value=[-0.878681374026269335075767230591736733913421630859375;1.2259935692682997210312123570474795997142791748046875;-0.30483174186242223413501051254570484161376953125;-1.4126017657634808433186890397337265312671661376953125;-0.16851205718232054042715617470094002783298492431640625;-0.90442286536734428636918892152607440948486328125;1.169452539822338099639864594792015850543975830078125]
      mask Display: e = 0.06;c1 = [120 150 230]/255;c2 = ([120 150 230]+0)/383;c3 = ([120 150 230]+128)/383;patch([0 1 1 0],[0 0 1 1],c1);patch([0 1 1 1-e 1-e 0+e],[0 0 1 1-e 0+e 0+e],c2);patch([0 0 1 1-e 0+e 0+e],[0 1 1 1-e 1-e 0+e],c3);plot([0 1 1 0 0],[0 0 1 1 0]);disp('Weights');
  "IW{1,1}(55,:)'" : Constant  Value=[0.08657117739125146094192331247541005723178386688232421875;1.55525590350724041144303555483929812908172607421875;1.571275680166724253439269887167029082775115966796875;0.0389356200283746123336214850496617145836353302001953125;1.0608030005091400038708115971530787646770477294921875;-0.1770242286839346645965775906006456352770328521728515625;0.8749463130276551314778998857946135103702545166015625]
      mask Display: e = 0.06;c1 = [120 150 230]/255;c2 = ([120 150 230]+0)/383;c3 = ([120 150 230]+128)/383;patch([0 1 1 0],[0 0 1 1],c1);patch([0 1 1 1-e 1-e 0+e],[0 0 1 1-e 0+e 0+e],c2);patch([0 0 1 1-e 0+e 0+e],[0 1 1 1-e 1-e 0+e],c3);plot([0 1 1 0 0],[0 0 1 1 0]);disp('Weights');
  "IW{1,1}(56,:)'" : Constant  Value=[1.237542557784059749081961854244582355022430419921875;-0.7639115927886688250936231270316056907176971435546875;0.74476614556811415734927095400053076446056365966796875;0.56954566336828893469146350980736315250396728515625;0.61565589059907599445153891792870126664638519287109375;-0.5376764926956756340814536088146269321441650390625;1.626904678049955865759557127603329718112945556640625]
      mask Display: e = 0.06;c1 = [120 150 230]/255;c2 = ([120 150 230]+0)/383;c3 = ([120 150 230]+128)/383;patch([0 1 1 0],[0 0 1 1],c1);patch([0 1 1 1-e 1-e 0+e],[0 0 1 1-e 0+e 0+e],c2);patch([0 0 1 1-e 0+e 0+e],[0 1 1 1-e 1-e 0+e],c3);plot([0 1 1 0 0],[0 0 1 1 0]);disp('Weights');
  "IW{1,1}(57,:)'" : Constant  Value=[-0.868078569057733062663828604854643344879150390625;-1.165974491241934973828620059066452085971832275390625;0.10609840146620587442161109947846853174269199371337890625;-0.90156681825631268534237960921018384397029876708984375;-2.428906126398517439923807614832185208797454833984375;0.73891351686324713288200882743694819509983062744140625;0.284503194421066918362583919588360004127025604248046875]
      mask Display: e = 0.06;c1 = [120 150 230]/255;c2 = ([120 150 230]+0)/383;c3 = ([120 150 230]+128)/383;patch([0 1 1 0],[0 0 1 1],c1);patch([0 1 1 1-e 1-e 0+e],[0 0 1 1-e 0+e 0+e],c2);patch([0 0 1 1-e 0+e 0+e],[0 1 1 1-e 1-e 0+e],c3);plot([0 1 1 0 0],[0 0 1 1 0]);disp('Weights');
  "IW{1,1}(58,:)'" : Constant  Value=[-1.30510909203312674975450136116705834865570068359375;-0.1671177331211633199092858603762579150497913360595703125;0.7358137655288110590134920130367390811443328857421875;1.501410257805670056541202939115464687347412109375;0.4089546848156242475624821963720023632049560546875;0.2678825310125543257555591480922885239124298095703125;-1.28614728448410264860513052553869783878326416015625]
      mask Display: e = 0.06;c1 = [120 150 230]/255;c2 = ([120 150 230]+0)/383;c3 = ([120 150 230]+128)/383;patch([0 1 1 0],[0 0 1 1],c1);patch([0 1 1 1-e 1-e 0+e],[0 0 1 1-e 0+e 0+e],c2);patch([0 0 1 1-e 0+e 0+e],[0 1 1 1-e 1-e 0+e],c3);plot([0 1 1 0 0],[0 0 1 1 0]);disp('Weights');
  "IW{1,1}(59,:)'" : Constant  Value=[0.78819067391595998284259394495165906846523284912109375;1.0049970900971356702058301380020566284656524658203125;1.7128181762409686594850199981010518968105316162109375;0.48388259774764652565437472730991430580615997314453125;0.6422572407911018022019788986654020845890045166015625;0.16319232352850365774799001883366145193576812744140625;-1.26925895141153954881474419380538165569305419921875]
      mask Display: e = 0.06;c1 = [120 150 230]/255;c2 = ([120 150 230]+0)/383;c3 = ([120 150 230]+128)/383;patch([0 1 1 0],[0 0 1 1],c1);patch([0 1 1 1-e 1-e 0+e],[0 0 1 1-e 0+e 0+e],c2);patch([0 0 1 1-e 0+e 0+e],[0 1 1 1-e 1-e 0+e],c3);plot([0 1 1 0 0],[0 0 1 1 0]);disp('Weights');
  "IW{1,1}(6,:)'" : Constant  Value=[-0.0677528317986960948449137731586233712732791900634765625;-1.504169779309772803088662840309552848339080810546875;-0.87929157452727857435803571206633932888507843017578125;-0.8760369945765915655755406987736932933330535888671875;-1.672337522207133719831517737475223839282989501953125;-1.4356226151765103526969369340804405510425567626953125;0.1592425066398253374888582811763626523315906524658203125]
      mask Display: e = 0.06;c1 = [120 150 230]/255;c2 = ([120 150 230]+0)/383;c3 = ([120 150 230]+128)/383;patch([0 1 1 0],[0 0 1 1],c1);patch([0 1 1 1-e 1-e 0+e],[0 0 1 1-e 0+e 0+e],c2);patch([0 0 1 1-e 0+e 0+e],[0 1 1 1-e 1-e 0+e],c3);plot([0 1 1 0 0],[0 0 1 1 0]);disp('Weights');
  "IW{1,1}(60,:)'" : Constant  Value=[-1.0722466703029087664589269479620270431041717529296875;0.73890371942793120485504232419771142303943634033203125;-1.9138338837816533111180206105927936732769012451171875;1.0277109431222444246856184690841473639011383056640625;0.2225103902039953507330238835493219085037708282470703125;0.420305641965908305390797750078490935266017913818359375;-0.320595525674717218844733679361524991691112518310546875]
      mask Display: e = 0.06;c1 = [120 150 230]/255;c2 = ([120 150 230]+0)/383;c3 = ([120 150 230]+128)/383;patch([0 1 1 0],[0 0 1 1],c1);patch([0 1 1 1-e 1-e 0+e],[0 0 1 1-e 0+e 0+e],c2);patch([0 0 1 1-e 0+e 0+e],[0 1 1 1-e 1-e 0+e],c3);plot([0 1 1 0 0],[0 0 1 1 0]);disp('Weights');
  "IW{1,1}(61,:)'" : Constant  Value=[0.51212952866549787955818828777410089969635009765625;-0.41556978307366587710447447534534148871898651123046875;-1.46597023740784759837652018177323043346405029296875;0.9822186865382089848708346835337579250335693359375;-0.7957700769446327537792740258737467229366302490234375;0.66162899620550075230340780763071961700916290283203125;-0.99999288616506809557193946602637879550457000732421875]
      mask Display: e = 0.06;c1 = [120 150 230]/255;c2 = ([120 150 230]+0)/383;c3 = ([120 150 230]+128)/383;patch([0 1 1 0],[0 0 1 1],c1);patch([0 1 1 1-e 1-e 0+e],[0 0 1 1-e 0+e 0+e],c2);patch([0 0 1 1-e 0+e 0+e],[0 1 1 1-e 1-e 0+e],c3);plot([0 1 1 0 0],[0 0 1 1 0]);disp('Weights');
  "IW{1,1}(62,:)'" : Constant  Value=[-9.3499717686009926609358444693498313426971435546875;-1.6687740105111006361227055094786919653415679931640625;0.3889865892122232882144317045458592474460601806640625;0.1628038449518091901335736793043906800448894500732421875;-2.078334660366574215828450178378261625766754150390625;-0.46747409568921749478676019862177781760692596435546875;0.68559383251914118861947144978330470621585845947265625]
      mask Display: e = 0.06;c1 = [120 150 230]/255;c2 = ([120 150 230]+0)/383;c3 = ([120 150 230]+128)/383;patch([0 1 1 0],[0 0 1 1],c1);patch([0 1 1 1-e 1-e 0+e],[0 0 1 1-e 0+e 0+e],c2);patch([0 0 1 1-e 0+e 0+e],[0 1 1 1-e 1-e 0+e],c3);plot([0 1 1 0 0],[0 0 1 1 0]);disp('Weights');
  "IW{1,1}(63,:)'" : Constant  Value=[1.3920560485040416320856593301868997514247894287109375;1.2192749778278735295344858968746848404407501220703125;-1.131174831914206979632808725000359117984771728515625;-0.72964851174637235242670385559904389083385467529296875;2.681255093203409156643601818359456956386566162109375;0.1257455976156408306021461385171278379857540130615234375;1.1240837671880845594074571636156179010868072509765625]
      mask Display: e = 0.06;c1 = [120 150 230]/255;c2 = ([120 150 230]+0)/383;c3 = ([120 150 230]+128)/383;patch([0 1 1 0],[0 0 1 1],c1);patch([0 1 1 1-e 1-e 0+e],[0 0 1 1-e 0+e 0+e],c2);patch([0 0 1 1-e 0+e 0+e],[0 1 1 1-e 1-e 0+e],c3);plot([0 1 1 0 0],[0 0 1 1 0]);disp('Weights');
  "IW{1,1}(64,:)'" : Constant  Value=[-1.1245895891605266481150238178088329732418060302734375;0.99216305797861503723567011547856964170932769775390625;1.216170922417554312033871610765345394611358642578125;1.00388928404632071789137626183219254016876220703125;0.349604984180501732193846464724629186093807220458984375;-0.36967499856060503926613591829664073884487152099609375;1.322827801452259421921553439460694789886474609375]
      mask Display: e = 0.06;c1 = [120 150 230]/255;c2 = ([120 150 230]+0)/383;c3 = ([120 150 230]+128)/383;patch([0 1 1 0],[0 0 1 1],c1);patch([0 1 1 1-e 1-e 0+e],[0 0 1 1-e 0+e 0+e],c2);patch([0 0 1 1-e 0+e 0+e],[0 1 1 1-e 1-e 0+e],c3);plot([0 1 1 0 0],[0 0 1 1 0]);disp('Weights');
  "IW{1,1}(7,:)'" : Constant  Value=[0.88358071509059088466386810978292487561702728271484375;-0.2349270917167734229469289175540325231850147247314453125;0.1366099851058469039077891693523270078003406524658203125;1.4171073584098905495665121634374372661113739013671875;0.96214074180150976900449677486903965473175048828125;-0.84241315143091222150673047508462332189083099365234375;1.1132897258254084160711272488697431981563568115234375]
      mask Display: e = 0.06;c1 = [120 150 230]/255;c2 = ([120 150 230]+0)/383;c3 = ([120 150 230]+128)/383;patch([0 1 1 0],[0 0 1 1],c1);patch([0 1 1 1-e 1-e 0+e],[0 0 1 1-e 0+e 0+e],c2);patch([0 0 1 1-e 0+e 0+e],[0 1 1 1-e 1-e 0+e],c3);plot([0 1 1 0 0],[0 0 1 1 0]);disp('Weights');
  "IW{1,1}(8,:)'" : Constant  Value=[-1.395733659940647353181475409655831754207611083984375;1.2086164758276940478509686727193184196949005126953125;-0.1732703398751260781551764011965133249759674072265625;0.93793237375914928488640498471795581281185150146484375;-1.0349425891455099613125412361114285886287689208984375;1.4481824947271686454541850253008306026458740234375;-0.188168293001181263779386654277914203703403472900390625]
      mask Display: e = 0.06;c1 = [120 150 230]/255;c2 = ([120 150 230]+0)/383;c3 = ([120 150 230]+128)/383;patch([0 1 1 0],[0 0 1 1],c1);patch([0 1 1 1-e 1-e 0+e],[0 0 1 1-e 0+e 0+e],c2);patch([0 0 1 1-e 0+e 0+e],[0 1 1 1-e 1-e 0+e],c3);plot([0 1 1 0 0],[0 0 1 1 0]);disp('Weights');
  "IW{1,1}(9,:)'" : Constant  Value=[-0.228720071439284355907517465311684645712375640869140625;-1.21806659245520076950697330175898969173431396484375;1.4189117114977516376228550143423490226268768310546875;0.5481062594804633203438015698338858783245086669921875;0.4298419096351138168898842195631004869937896728515625;1.4680607869905344387007062323391437530517578125;-0.409392364118598084399280878642457537353038787841796875]
      mask Display: e = 0.06;c1 = [120 150 230]/255;c2 = ([120 150 230]+0)/383;c3 = ([120 150 230]+128)/383;patch([0 1 1 0],[0 0 1 1],c1);patch([0 1 1 1-e 1-e 0+e],[0 0 1 1-e 0+e 0+e],c2);patch([0 0 1 1-e 0+e 0+e],[0 1 1 1-e 1-e 0+e],c3);plot([0 1 1 0 0],[0 0 1 1 0]);disp('Weights');
  Mux : Mux  Inputs=64
      mask Display: e = 0.06;c1 = [120 150 230]/255;c2 = ([120 150 230]+0)/383;c3 = ([120 150 230]+128)/383;patch([0 1 1 0],[0 0 1 1],c1);patch([0 1 1 1-e 1-e 0+e],[0 0 1 1-e 0+e 0+e],c2);patch([0 0 1 1-e 0+e 0+e],[0 1 1 1-e 1-e 0+e],c3);plot([0 1 1 0 0],[0 0 1 1 0]);disp('Mux');
  dotprod{1..64} (64 alike) : neural/Weight Functions/dotprod
  "iz{1,1}" : Outport
      mask Display: e = 0.06;c1 = [120 230 180]/255;c2 = ([120 230 180]+0)/(256+128);c3 = ([120 230 180]+128)/(256+128);patch([0 1 1 0],[0 0 1 1],c1);patch([0 1 1 1-e 1-e 0+e],[0 0 1 1-e 0+e 0+e],c2);patch([0 0 1 1-e 0+e 0+e],[0 1 1 1-e 1-e 0+e],c3);plot([0 1 1 0 0],[0 0 1 1 0]);
  wires:
  "IW{1,1}(1,:)'"/1 -> dotprod1/1
  "pd{1,1}"/1 -> dotprod1/2, dotprod2/2, dotprod3/2, dotprod4/2, dotprod5/2, dotprod6/2, dotprod7/2, dotprod8/2, dotprod9/2, dotprod10/2, dotprod11/2, dotprod12/2, dotprod13/2, dotprod14/2, dotprod15/2, dotprod16/2, dotprod17/2, dotprod18/2, dotprod19/2, dotprod20/2, dotprod21/2, dotprod22/2, dotprod23/2, dotprod24/2, dotprod25/2, dotprod26/2, dotprod27/2, dotprod28/2, dotprod29/2, dotprod30/2, dotprod31/2, dotprod32/2, dotprod33/2, dotprod34/2, dotprod35/2, dotprod36/2, dotprod37/2, dotprod38/2, dotprod39/2, dotprod40/2, dotprod41/2, dotprod42/2, dotprod43/2, dotprod44/2, dotprod45/2, dotprod46/2, dotprod47/2, dotprod48/2, dotprod49/2, dotprod50/2, dotprod51/2, dotprod52/2, dotprod53/2, dotprod54/2, dotprod55/2, dotprod56/2, dotprod57/2, dotprod58/2, dotprod59/2, dotprod60/2, dotprod61/2, dotprod62/2, dotprod63/2, dotprod64/2
  dotprod1/1 -> Mux/1
  "IW{1,1}(2,:)'"/1 -> dotprod2/1
  dotprod2/1 -> Mux/2
  "IW{1,1}(3,:)'"/1 -> dotprod3/1
  dotprod3/1 -> Mux/3
  "IW{1,1}(4,:)'"/1 -> dotprod4/1
  dotprod4/1 -> Mux/4
  "IW{1,1}(5,:)'"/1 -> dotprod5/1
  dotprod5/1 -> Mux/5
  "IW{1,1}(6,:)'"/1 -> dotprod6/1
  dotprod6/1 -> Mux/6
  "IW{1,1}(7,:)'"/1 -> dotprod7/1
  dotprod7/1 -> Mux/7
  "IW{1,1}(8,:)'"/1 -> dotprod8/1
  dotprod8/1 -> Mux/8
  "IW{1,1}(9,:)'"/1 -> dotprod9/1
  dotprod9/1 -> Mux/9
  "IW{1,1}(10,:)'"/1 -> dotprod10/1
  dotprod10/1 -> Mux/10
  "IW{1,1}(11,:)'"/1 -> dotprod11/1
  dotprod11/1 -> Mux/11
  "IW{1,1}(12,:)'"/1 -> dotprod12/1
  dotprod12/1 -> Mux/12
  "IW{1,1}(13,:)'"/1 -> dotprod13/1
  dotprod13/1 -> Mux/13
  "IW{1,1}(14,:)'"/1 -> dotprod14/1
  dotprod14/1 -> Mux/14
  "IW{1,1}(15,:)'"/1 -> dotprod15/1
  dotprod15/1 -> Mux/15
  "IW{1,1}(16,:)'"/1 -> dotprod16/1
  dotprod16/1 -> Mux/16
  "IW{1,1}(17,:)'"/1 -> dotprod17/1
  dotprod17/1 -> Mux/17
  "IW{1,1}(18,:)'"/1 -> dotprod18/1
  dotprod18/1 -> Mux/18
  "IW{1,1}(19,:)'"/1 -> dotprod19/1
  dotprod19/1 -> Mux/19
  "IW{1,1}(20,:)'"/1 -> dotprod20/1
  dotprod20/1 -> Mux/20
  "IW{1,1}(21,:)'"/1 -> dotprod21/1
  dotprod21/1 -> Mux/21
  "IW{1,1}(22,:)'"/1 -> dotprod22/1
  dotprod22/1 -> Mux/22
  "IW{1,1}(23,:)'"/1 -> dotprod23/1
  dotprod23/1 -> Mux/23
  "IW{1,1}(24,:)'"/1 -> dotprod24/1
  dotprod24/1 -> Mux/24
  "IW{1,1}(25,:)'"/1 -> dotprod25/1
  dotprod25/1 -> Mux/25
  "IW{1,1}(26,:)'"/1 -> dotprod26/1
  dotprod26/1 -> Mux/26
  "IW{1,1}(27,:)'"/1 -> dotprod27/1
  dotprod27/1 -> Mux/27
  "IW{1,1}(28,:)'"/1 -> dotprod28/1
  dotprod28/1 -> Mux/28
  "IW{1,1}(29,:)'"/1 -> dotprod29/1
  dotprod29/1 -> Mux/29
  "IW{1,1}(30,:)'"/1 -> dotprod30/1
  dotprod30/1 -> Mux/30
  "IW{1,1}(31,:)'"/1 -> dotprod31/1
  dotprod31/1 -> Mux/31
  "IW{1,1}(32,:)'"/1 -> dotprod32/1
  dotprod32/1 -> Mux/32
  "IW{1,1}(33,:)'"/1 -> dotprod33/1
  dotprod33/1 -> Mux/33
  "IW{1,1}(34,:)'"/1 -> dotprod34/1
  dotprod34/1 -> Mux/34
  "IW{1,1}(35,:)'"/1 -> dotprod35/1
  dotprod35/1 -> Mux/35
  "IW{1,1}(36,:)'"/1 -> dotprod36/1
  dotprod36/1 -> Mux/36
  "IW{1,1}(37,:)'"/1 -> dotprod37/1
  dotprod37/1 -> Mux/37
  "IW{1,1}(38,:)'"/1 -> dotprod38/1
  dotprod38/1 -> Mux/38
  "IW{1,1}(39,:)'"/1 -> dotprod39/1
  dotprod39/1 -> Mux/39
  "IW{1,1}(40,:)'"/1 -> dotprod40/1
  dotprod40/1 -> Mux/40
  "IW{1,1}(41,:)'"/1 -> dotprod41/1
  dotprod41/1 -> Mux/41
  "IW{1,1}(42,:)'"/1 -> dotprod42/1
  dotprod42/1 -> Mux/42
  "IW{1,1}(43,:)'"/1 -> dotprod43/1
  dotprod43/1 -> Mux/43
  "IW{1,1}(44,:)'"/1 -> dotprod44/1
  dotprod44/1 -> Mux/44
  "IW{1,1}(45,:)'"/1 -> dotprod45/1
  dotprod45/1 -> Mux/45
  "IW{1,1}(46,:)'"/1 -> dotprod46/1
  dotprod46/1 -> Mux/46
  "IW{1,1}(47,:)'"/1 -> dotprod47/1
  dotprod47/1 -> Mux/47
  "IW{1,1}(48,:)'"/1 -> dotprod48/1
  dotprod48/1 -> Mux/48
  "IW{1,1}(49,:)'"/1 -> dotprod49/1
  dotprod49/1 -> Mux/49
  "IW{1,1}(50,:)'"/1 -> dotprod50/1
  dotprod50/1 -> Mux/50
  "IW{1,1}(51,:)'"/1 -> dotprod51/1
  dotprod51/1 -> Mux/51
  "IW{1,1}(52,:)'"/1 -> dotprod52/1
  dotprod52/1 -> Mux/52
  "IW{1,1}(53,:)'"/1 -> dotprod53/1
  dotprod53/1 -> Mux/53
  "IW{1,1}(54,:)'"/1 -> dotprod54/1
  dotprod54/1 -> Mux/54
  "IW{1,1}(55,:)'"/1 -> dotprod55/1
  dotprod55/1 -> Mux/55
  "IW{1,1}(56,:)'"/1 -> dotprod56/1
  dotprod56/1 -> Mux/56
  "IW{1,1}(57,:)'"/1 -> dotprod57/1
  dotprod57/1 -> Mux/57
  "IW{1,1}(58,:)'"/1 -> dotprod58/1
  dotprod58/1 -> Mux/58
  "IW{1,1}(59,:)'"/1 -> dotprod59/1
  dotprod59/1 -> Mux/59
  "IW{1,1}(60,:)'"/1 -> dotprod60/1
  dotprod60/1 -> Mux/60
  "IW{1,1}(61,:)'"/1 -> dotprod61/1
  dotprod61/1 -> Mux/61
  "IW{1,1}(62,:)'"/1 -> dotprod62/1
  dotprod62/1 -> Mux/62
  "IW{1,1}(63,:)'"/1 -> dotprod63/1
  dotprod63/1 -> Mux/63
  "IW{1,1}(64,:)'"/1 -> dotprod64/1
  dotprod64/1 -> Mux/64
  Mux/1 -> "iz{1,1}"/1
